simulink model "atherton_lab_1"  (R2018a)
settings: Solver=ode23t  StartTime=0.0  StopTime=20  RelTol=1e-3
settings Model: Creator=katherto  LastModifiedBy=katherto

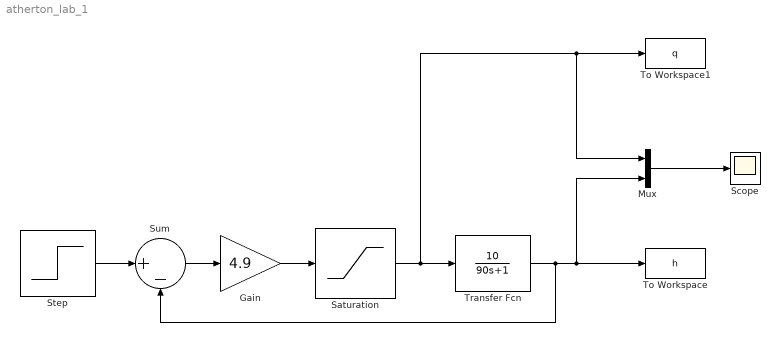
== system atherton_lab_1 ==
  Gain : Gain  Gain=4.9
  Mux : Mux  Inputs=2
  Saturation : Saturate  UpperLimit=1  LowerLimit=0
  Scope : Scope
  Step : Step  Time=0  SampleTime=0
  Sum : Sum  Inputs=|+-
  To Workspace : ToWorkspace  VariableName=h  SaveFormat=Timeseries  SampleTime=-1
  To Workspace1 : ToWorkspace  VariableName=q  SaveFormat=Timeseries  SampleTime=-1
  Transfer Fcn : TransferFcn  Numerator=10  Denominator=[90 1]
  wires:
  Step/1 -> Sum/1
  Sum/1 -> Gain/1
  Gain/1 -> Saturation/1
  Saturation/1 -> Mux/1, To Workspace1/1, Transfer Fcn/1
  Transfer Fcn/1 -> Sum/2, Mux/2, To Workspace/1
  Mux/1 -> Scope/1
